simulink model "ADC"  (R2015a)
settings: Solver=ode45  StartTime=0.0  StopTime=10e-5  RelTol=1e-3
libraries: dsparch4 x1
settings Model: Creator=John  LastModifiedBy=John

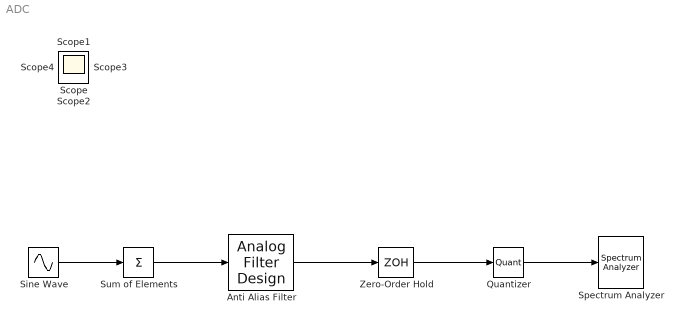
== system ADC ==
  "Anti Alias Filter " : dsparch4/Analog Filter Design  method=Butterworth  filttype=Lowpass  N=8  Wlo=2*pi*50e6  Whi=80  Rp=2  Rs=40
  Quantizer : Quantizer  QuantizationInterval=2^-8
  Sine Wave : Sin  Amplitude=.25  Frequency=2*pi*[20 21 22 23]*1e6  SampleTime=0
  "Spectrum Analyzer " : SpectrumAnalyzer
  Sum of Elements : Sum  Inputs=+
  Zero-Order Hold : ZeroOrderHold  SampleTime=1/100e6
  Scope{,1..4} (5 alike) : Scope
      Scope settings: TimeRange=2.060541768966431e-07  YMin=-0.25  YMax=0.25
      Scope1 settings: TimeRange=3.018355235392037e-06  YMin=-0.5  YMax=0.5
      Scope2 settings: TimeRange=3.37060150351322e-06  YMin=-0.5  YMax=0.5  SaveName=ScopeData2
      Scope3 settings: TimeRange=2.972373570352188e-06  YMin=-0.5  YMax=0.5  SaveName=ScopeData3
      Scope4 settings: SaveName=ScopeData4
  wires:
  Sine Wave/1 -> Sum of Elements/1
  Sum of Elements/1 -> "Anti Alias Filter "/1
  "Anti Alias Filter "/1 -> Zero-Order Hold/1
  Zero-Order Hold/1 -> Quantizer/1
  Quantizer/1 -> "Spectrum Analyzer "/1
